simulink model "SimulinkModel"  (R2023a)
settings: Solver=FixedStepAuto  StartTime=0.0  StopTime=TimeSpan  FixedStep=DT  RelTol=1e-3
values from neighbouring files (symbols this model uses):
  A = [0 1 0 0 0 ... (first row only)    [Main.m]    (also in SweepTest.m; myActiveSuspensions.mat = [0 -861.462979483 0 763.157894737 0 1 -89.1168599465 0 78.94)
  AO = A-KO*C    [Main.m]    (also in SweepTest.m; myActiveSuspensions.mat = [-6.29015203402 -9209.07677924 -1030.51480744 -503585.757509)
  B1 = [0;0;0;0;mi*gamma*sqrt(Ps/rho)]    [Main.m]    (also in SweepTest.m = [0;0;0;0;mi*gamma]; myActiveSuspensions.mat = [0 0 0 0 154.5])
  B2 = [0 0 0 0 0 0 ... (first row only)    [Main.m]    (also in SweepTest.m; myActiveSuspensions.mat = [0 0 0 -1 0 0 0.00338983050847 0 0 0 0 0 ... (30 elements, 5)
  BO = B1-KO*D1    [Main.m]    (also in SweepTest.m; myActiveSuspensions.mat = [0 0 0 0 154.5])
  C = [1 0 0 0 0 ... (first row only)    [Main.m]    (also in SweepTest.m; myActiveSuspensions.mat = [1 1 -98.3050847458 0 0 -10.1694915254 0 1 0 0 0 0 ... (15 e)
  Ce = [1 0 0 0 0]    [Main.m]    (also in SweepTest.m; myActiveSuspensions.mat)
  Ceps = [1 0 0 0 0 0 ... (first row only)    [Main.m]    (also in SweepTest.m; myActiveSuspensions.mat = [1 0 0 0 0 0 -98.3050847458 1 0 1 0 0 ... (48 elements, 8x6))
  CO = eye(n)    [Main.m]    (also in SweepTest.m; myActiveSuspensions.mat = [1 0 0 0 0 0 1 0 0 0 0 0 ... (25 elements, 5x5)])
  D1 = [0;0;0]    [Main.m]    (also in SweepTest.m; myActiveSuspensions.mat = [0 0 0])
  D2 = [0 0 1 0 0 0 ... (first row only)    [Main.m]    (also in SweepTest.m; myActiveSuspensions.mat = [0 0 0 0 0 0.00338983050847 1 0 0 0 1 0 ... (18 elements, 3x)
  De1 = [0]    [Main.m]    (also in SweepTest.m = 0; myActiveSuspensions.mat = 0)
  De2 = [0 0 1 0 0 -1]    [Main.m]    (also in SweepTest.m; myActiveSuspensions.mat)
  drive_mode = 0    [Main.m]    (also in SweepTest.m; myActiveSuspensions.mat = 2)
  DT = 1e-3    (= 0.001)    [Main.m]    (also in SweepTest.m = 0.0001; myActiveSuspensions.mat = 0.0001)
  e0 = [y0(3) ... (first row only)    [Main.m]    (also in SweepTest.m = y0(1) - r0; myActiveSuspensions.mat = 0)
  KI = K(:,n+1:n+m)    [Main.m]    (also in SweepTest.m; myActiveSuspensions.mat = -14142.1356237)
  KO = Km.'    [Main.m]    (also in SweepTest.m; myActiveSuspensions.mat = [0.176588896427 58.0307081184 2.94746555023 -226.466108515 -)
  KS = K(:,1:n)    [Main.m]    (also in SweepTest.m; myActiveSuspensions.mat = [-6270.88767395 -1376.60013396 -1626.06750459 -11.6411551471)
  m = 1    [Main.m]    (also in SweepTest.m; myActiveSuspensions.mat)
  n = size(V)    [JCF.m]    (also in Main.m = 5; SweepTest.m = 5; myActiveSuspensions.mat = 5)
  p = 1    [Main.m]    (also in SweepTest.m; myActiveSuspensions.mat)
  q = length(index{i})    [JCF.m]    (also in Main.m = 3; SweepTest.m = 3; myActiveSuspensions.mat = 3)
  r = nd + q + m    (= 6)    [Main.m]    (also in SweepTest.m; myActiveSuspensions.mat)
  u0 = 0    [Main.m]    (also in SweepTest.m; myActiveSuspensions.mat)
  w0 = [d0; nu0; r0]    [Main.m]    (also in SweepTest.m; myActiveSuspensions.mat = [0 -91.875 0 0 0 0.597040517241])
  x0 = [l0s-g*ms/ks ... (first row only)    [Main.m]    (also in SweepTest.m = [- g*ms/ks + l0s + Lift/ks; myActiveSuspensions.mat = [0.597040517241 0 0.3385371843 0 0])
  x_init = [zs_init-zu_init ... (first row only)    [Main.m]    (also in SweepTest.m = [(- g*ms/ks + l0s + Lift/ks) - Diseq; myActiveSuspensions.mat = [0.597040517241 0 0.3385371843 0 0])
  y0 = [x0(1) ... (first row only)    [Main.m]    (also in SweepTest.m; myActiveSuspensions.mat = [0.597040517241 0.935577701542 6.16606577473e-15])
undefined symbols (not defined in the file or in its folder): Deps, PLANT, scenario, tilde_x_init, xO_init
settings Model: Creator=nicola.mimmo2  LastModifiedBy=aleze
settings DebuggingCC: UnconnectedInputMsg=warning  UnconnectedOutputMsg=warning  UnconnectedLineMsg=warning
settings ModelReferenceCC: EnableRefExpFcnMdlSchedulingChecks=on
settings RTWCC: DLArmComputeVersion=19.05

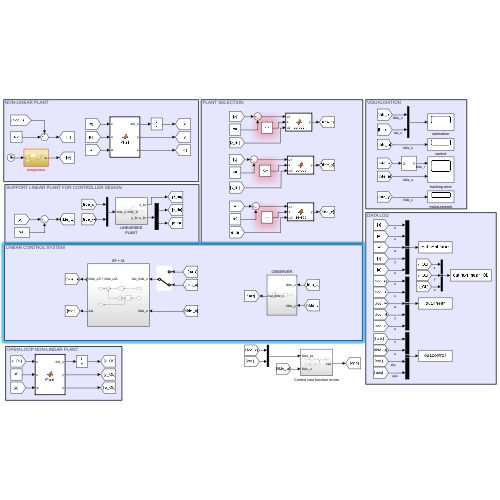
[thumbnail: Simulink's stored preview of the top-level diagram]
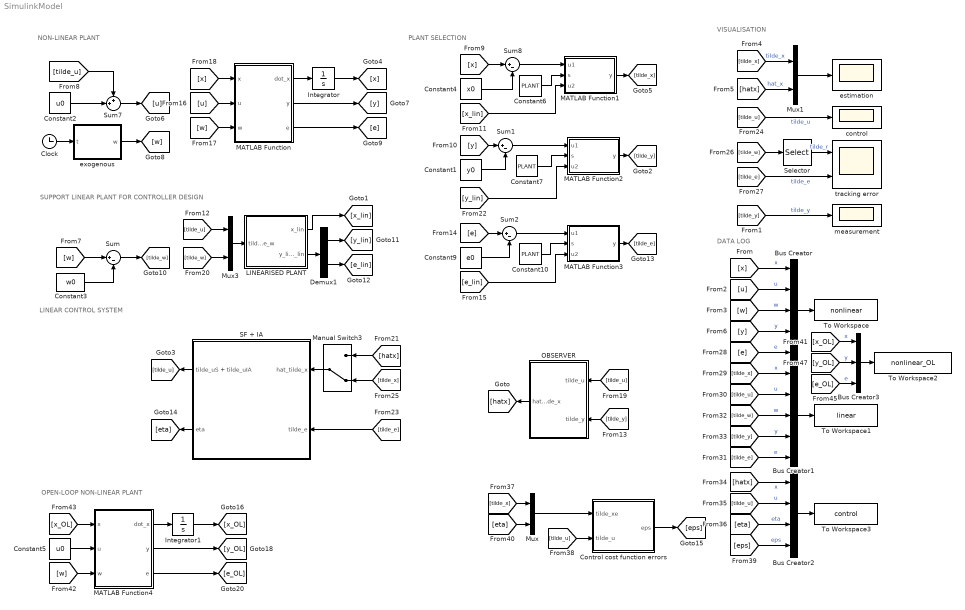
== system SimulinkModel ==
  note: DATA LOG
  note: VISUALISATION
  note: PLANT SELECTION
  note: NON-LINEAR PLANT
  note: SUPPORT LINEAR PLANT FOR CONTROLLER DESIGN
  note: LINEAR CONTROL SYSTEM
  note: OPEN-LOOP NON-LINEAR PLANT
  Bus Creator : BusCreator  Inputs=5
  Bus Creator1 : BusCreator  Inputs=5
  Bus Creator2 : BusCreator  Inputs=4
  Bus Creator3 : BusCreator  Inputs=3
  Clock : Clock
  Constant1 : Constant  Value=y0
  Constant10 : Constant  Value=PLANT
  Constant2 : Constant  Value=u0
  Constant3 : Constant  Value=w0
  Constant4 : Constant  Value=x0
  Constant5 : Constant  Value=u0
  Constant6 : Constant  Value=PLANT
  Constant7 : Constant  Value=PLANT
  Constant9 : Constant  Value=e0
  Control cost function errors : Subsystem
  Demux1 : Demux  Outputs=[q m]
  Integrator : Integrator  InitialCondition=x_init
  Integrator1 : Integrator  InitialCondition=x_init
  LINEARISED PLANT : Subsystem
  MATLAB Function : MATLAB Function  TreatAsAtomicUnit=on
  MATLAB Function1 : MATLAB Function  TreatAsAtomicUnit=on
  MATLAB Function2 : MATLAB Function  TreatAsAtomicUnit=on
  MATLAB Function3 : MATLAB Function  TreatAsAtomicUnit=on
  MATLAB Function4 : MATLAB Function  TreatAsAtomicUnit=on
  Manual Switch3 : ManualSwitch  CurrentSetting=0
  Mux : Mux  Inputs=2
  Mux1 : Mux  Inputs=2
  Mux3 : Mux  Inputs=2
  OBSERVER : Subsystem
  SF + IA : Subsystem
  Selector : Selector  InputPortWidth=r  IndexOptions=Index vector (dialog)  Indices=[r-m+1:1:r]  OutputSizes=1
  Sum{,1..2,8} (4 alike) : Sum  Inputs=|+-
  Sum7 : Sum  Inputs=++|
  To Workspace : ToWorkspace  VariableName=nonlinear  SaveFormat=Timeseries  SampleTime=-1
  To Workspace1 : ToWorkspace  VariableName=linear  SaveFormat=Timeseries  SampleTime=-1
  To Workspace2 : ToWorkspace  VariableName=nonlinear_OL  SaveFormat=Timeseries  SampleTime=-1
  To Workspace3 : ToWorkspace  VariableName=control  SaveFormat=Timeseries  SampleTime=-1
  control : Scope
  estimation : Scope
  exogenous : Subsystem
  measurement : Scope
  tracking error : Scope  NumInputPorts=2
  wires:
  Integrator/1 -> [x]
  Constant3/1 -> Sum/2
  Mux3/1 -> LINEARISED PLANT/1(tilde_u tilde_w)
  OBSERVER/1(hat_tilde_x) -> [hatx]
  [tilde_x] -> Mux1/1  "tilde_x"
  [hatx] -> Mux1/2  "hat_x"
  SF + IA/1(tilde_uS + tilde_uIA) -> [tilde_u]
  Constant2/1 -> Sum7/2
  Sum7/1 -> [u]
  [tilde_u] -> Sum7/1
  Constant1/1 -> Sum1/2
  Sum1/1 -> MATLAB Function2/1(u1)
  [y] -> Sum1/1
  [w] -> Sum/1
  [x] -> Sum8/1
  Constant4/1 -> Sum8/2
  Sum8/1 -> MATLAB Function1/1(u1)
  [x_lin] -> MATLAB Function1/3(u2)
  [tilde_e] -> SF + IA/2(tilde_e)
  [tilde_u] -> Mux3/1
  [u] -> MATLAB Function/2(u)
  [w] -> MATLAB Function/3(w)
  [x] -> MATLAB Function/1(x)
  Sum/1 -> [tilde_w]
  [tilde_w] -> Mux3/2
  [y_lin] -> MATLAB Function2/3(u2)
  Demux1/1 -> [y_lin]
  Demux1/2 -> [e_lin]
  [tilde_u] -> OBSERVER/1(tilde_u)
  Manual Switch3/1 -> SF + IA/1(hat_tilde_x)
  [hatx] -> Manual Switch3/1
  [tilde_x] -> Manual Switch3/2
  MATLAB Function/3(e) -> [e]
  MATLAB Function/2(y) -> [y]
  LINEARISED PLANT/1(x_lin) -> [x_lin]
  LINEARISED PLANT/2(y_lin e_lin) -> Demux1/1
  Clock/1 -> exogenous/1(t)
  exogenous/1(w) -> [w]
  MATLAB Function/1(dot_x) -> Integrator/1
  Mux1/1 -> estimation/1
  Constant6/1 -> MATLAB Function1/2(s)
  MATLAB Function1/1(y) -> [tilde_x]
  Constant7/1 -> MATLAB Function2/2(s)
  [tilde_y] -> OBSERVER/2(tilde_y)
  [e_lin] -> MATLAB Function3/3(u2)
  Constant9/1 -> Sum2/2
  Sum2/1 -> MATLAB Function3/1(u1)
  Constant10/1 -> MATLAB Function3/2(s)
  [e] -> Sum2/1
  [tilde_u] -> control/1  "tilde_u"
  [tilde_w] -> Selector/1
  Selector/1 -> tracking error/1  "tilde_r"
  [tilde_e] -> tracking error/2  "tilde_e"
  [tilde_y] -> measurement/1  "tilde_y"
  [y] -> Bus Creator/4  "y"
  [e] -> Bus Creator/5  "e"
  [w] -> Bus Creator/3  "w"
  [u] -> Bus Creator/2  "u"
  [x] -> Bus Creator/1  "x"
  Bus Creator/1 -> To Workspace/1
  [tilde_u] -> Bus Creator1/2  "u"
  [tilde_w] -> Bus Creator1/3  "w"
  [tilde_x] -> Bus Creator1/1  "x"
  [tilde_e] -> Bus Creator1/5  "e"
  [tilde_y] -> Bus Creator1/4  "y"
  Bus Creator1/1 -> To Workspace1/1
  SF + IA/2(eta) -> [eta]
  MATLAB Function2/1(y) -> [tilde_y]
  MATLAB Function3/1(y) -> [tilde_e]
  [hatx] -> Bus Creator2/1  "x"
  [tilde_u] -> Bus Creator2/2  "u"
  [eta] -> Bus Creator2/3  "eta"
  Bus Creator2/1 -> To Workspace3/1
  [tilde_u] -> Control cost function errors/2(tilde_u)
  Control cost function errors/1(eps) -> [eps]
  [eps] -> Bus Creator2/4  "eps"
  [tilde_x] -> Mux/1
  [eta] -> Mux/2
  Mux/1 -> Control cost function errors/1(tilde_xe)
  Integrator1/1 -> [x_OL]
  MATLAB Function4/3(e) -> [e_OL]
  MATLAB Function4/2(y) -> [y_OL]
  Constant5/1 -> MATLAB Function4/2(u)
  MATLAB Function4/1(dot_x) -> Integrator1/1
  [x_OL] -> MATLAB Function4/1(x)
  [w] -> MATLAB Function4/3(w)
  Bus Creator3/1 -> To Workspace2/1
  [x_OL] -> Bus Creator3/1  "x"
  [y_OL] -> Bus Creator3/2  "y"
  [e_OL] -> Bus Creator3/3  "e"

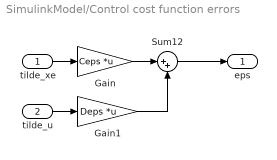
== system SimulinkModel/Control cost function errors ==
  tilde_xe : Inport
  tilde_u : Inport  Port=2
  Gain : Gain  Gain=Ceps  Multiplication=Matrix(K*u)
  Gain1 : Gain  Gain=Deps  Multiplication=Matrix(K*u)
  Sum12 : Sum  Inputs=|++
  eps : Outport
  wires:
  Gain1/1 -> Sum12/2
  Gain/1 -> Sum12/1
  Sum12/1 -> eps/1
  tilde_xe/1 -> Gain/1
  tilde_u/1 -> Gain1/1

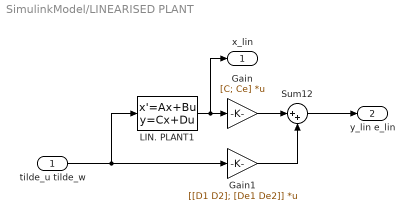
== system SimulinkModel/LINEARISED PLANT ==
  tilde_u tilde_w : Inport
  Gain : Gain  Gain=[C; Ce]  Multiplication=Matrix(K*u)
  Gain1 : Gain  Gain=[[D1 D2]; [De1 De2]]  Multiplication=Matrix(K*u)
  LIN. PLANT1 : StateSpace  A=A  B=[B1 B2]  C=eye(n)  D=zeros(n,p+r)  InitialCondition=tilde_x_init
  Sum12 : Sum  Inputs=|++
  x_lin : Outport
  y_lin e_lin : Outport  Port=2
  wires:
  Gain1/1 -> Sum12/2
  tilde_u tilde_w/1 -> Gain1/1, LIN. PLANT1/1
  Gain/1 -> Sum12/1
  LIN. PLANT1/1 -> x_lin/1, Gain/1
  Sum12/1 -> y_lin e_lin/1

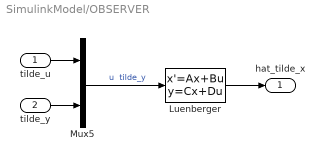
== system SimulinkModel/OBSERVER ==
  tilde_u : Inport
  tilde_y : Inport  Port=2
  Luenberger : StateSpace  A=AO  B=[BO KO]  C=CO  D=zeros(n,p+q)  InitialCondition=xO_init
  Mux5 : Mux  Inputs=2
  hat_tilde_x : Outport
  wires:
  tilde_u/1 -> Mux5/1
  Mux5/1 -> Luenberger/1  "u  tilde_y"
  tilde_y/1 -> Mux5/2
  Luenberger/1 -> hat_tilde_x/1

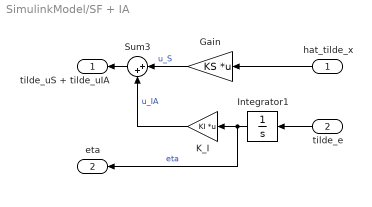
== system SimulinkModel/SF + IA ==
  hat_tilde_x : Inport
  tilde_e : Inport  Port=2
  Gain : Gain  Gain=KS  Multiplication=Matrix(K*u)
  Integrator1 : Integrator
  K_I : Gain  Gain=KI  Multiplication=Matrix(K*u)
  Sum3 : Sum  Inputs=|++
  tilde_uS + tilde_uIA : Outport
  eta : Outport  Port=2
  wires:
  Gain/1 -> Sum3/1  "u_S"
  Integrator1/1 -> eta/1, K_I/1  "eta"
  tilde_e/1 -> Integrator1/1
  K_I/1 -> Sum3/2  "u_IA"
  hat_tilde_x/1 -> Gain/1
  Sum3/1 -> tilde_uS + tilde_uIA/1

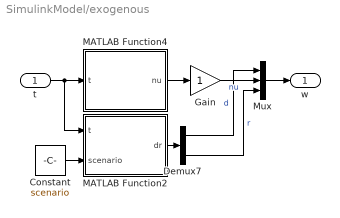
== system SimulinkModel/exogenous ==
  t : Inport
  Constant : Constant  Value=scenario
  Demux7 : Demux  Outputs=[1 1]
  Gain : Gain
  MATLAB Function2 : MATLAB Function  TreatAsAtomicUnit=on  mask{scenario=drive_mode}
      mask prompts: scenario "City, Race, Off-Road"
  MATLAB Function4 : MATLAB Function  TreatAsAtomicUnit=on  SystemSampleTime=DT
  Mux : Mux  Inputs=3
  w : Outport
  wires:
  Demux7/1 -> Mux/1  "d"
  Mux/1 -> w/1
  Demux7/2 -> Mux/3  "r"
  t/1 -> MATLAB Function2/1(t), MATLAB Function4/1(t)
  MATLAB Function2/1(dr) -> Demux7/1
  MATLAB Function4/1(nu) -> Gain/1
  Gain/1 -> Mux/2  "nu"
  Constant/1 -> MATLAB Function2/2(scenario)

== matlab function SimulinkModel/MATLAB Function1 ==
  data: u1 input; s input; y output; u2 input
function y = select(u1,s,u2)

if s == 0
    y = u2;
else
    y = u1;
end

== matlab function SimulinkModel/MATLAB Function ==
  data: x input; u input; dot_x output; w input; y output; e output
function [dot_x,y,e] = Plant(x,u,w)
[dot_x,y,e] = F(x,u,w);
end

== matlab function SimulinkModel/exogenous/MATLAB Function2 ==
  data: t input; dr output; scenario input
function dr = distANDref(t,scenario)

dr = [disturbance(t,scenario)
      reference(t,scenario)];

== matlab function SimulinkModel/MATLAB Function2 ==
  data: u1 input; s input; y output; u2 input
function y = select(u1,s,u2)

if s == 0
    y = u2;
else
    y = u1;
end

== matlab function SimulinkModel/exogenous/MATLAB Function4 ==
  data: t input; nu output
function nu = noises(t)

nu = noise(t);

== matlab function SimulinkModel/MATLAB Function3 ==
  data: u1 input; s input; y output; u2 input
function y = select(u1,s,u2)

if s == 0
    y = u2;
else
    y = u1;
end

== matlab function SimulinkModel/MATLAB Function4 ==
  data: x input; u input; dot_x output; w input; y output; e output
function [dot_x,y,e] = Plant(x,u,w)
[dot_x,y,e] = F(x,u,w);
end
